simulink model "MultipleAgentsChoice_NoVR"  (Simulink 7.5)
settings: Solver=ode45  StartTime=0.0  StopTime=1000  RelTol=1e-4  AbsTol=1e-4
libraries: simulink x64
(part 2 of 6)

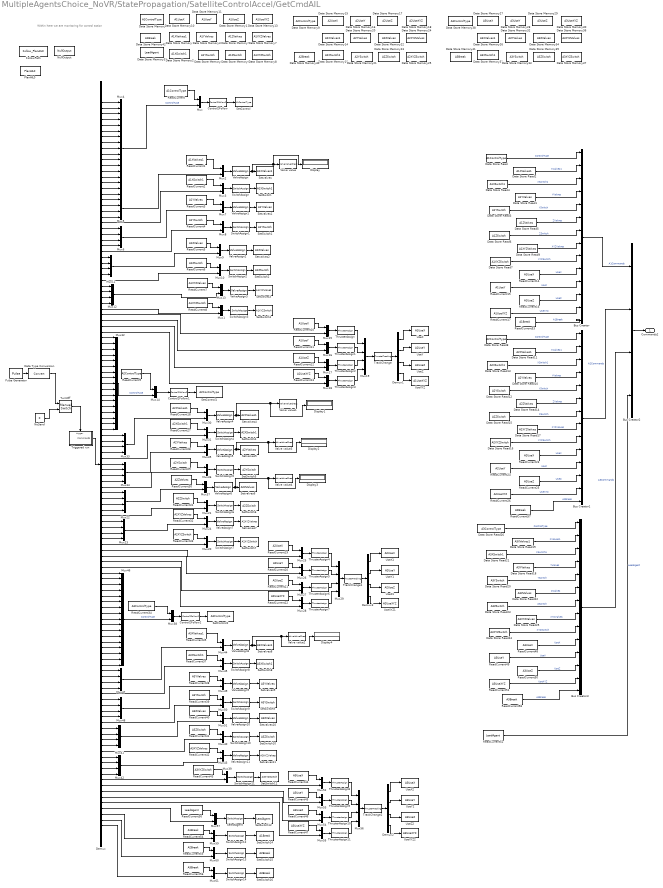
== system MultipleAgentsChoice_NoVR/StatePropagation/SatelliteControlAccel/GetCmdAIL ==
  note: Within here we are monitoring for control action
  Bus Creator : BusCreator  Inputs=14
  Bus Creator1 : BusCreator  Inputs=14
  Bus Creator2 : BusCreator
  Bus Creator3 : BusCreator  Inputs=14
  Control2Follow : MATLABFcn  MATLABFcn=Control2Follow2  OutputDimensions=17
  Control2Follow1 : MATLABFcn  MATLABFcn=Control2Follow2  OutputDimensions=17
  Control2Follow2 : MATLABFcn  MATLABFcn=Control2Follow2  OutputDimensions=17
  Data Store Memory : DataStoreMemory  DataStoreName=A1ControlType  ReadBeforeWriteMsg=warning  WriteAfterWriteMsg=warning  WriteAfterReadMsg=warning  InitialValue=[78;117;108;108;79;117;116;112;117;116;1;1;1;1;1;1;1]  OutDataType=sfix(16)  OutScaling=2^0
  Data Store Memory1 : DataStoreMemory  DataStoreName=A1XValves1  ReadBeforeWriteMsg=warning  WriteAfterWriteMsg=warning  WriteAfterReadMsg=warning  InitialValue=[2,2,1,1]  OutDataType=sfix(16)  OutScaling=2^0
  Data Store Memory10 : DataStoreMemory  DataStoreName=A1UseX  ReadBeforeWriteMsg=warning  WriteAfterWriteMsg=warning  WriteAfterReadMsg=warning  InitialValue=1  OutDataType=sfix(16)  OutScaling=2^0
  Data Store Memory11 : DataStoreMemory  DataStoreName=A1UseY  ReadBeforeWriteMsg=warning  WriteAfterWriteMsg=warning  WriteAfterReadMsg=warning  InitialValue=1  OutDataType=sfix(16)  OutScaling=2^0
  Data Store Memory12 : DataStoreMemory  DataStoreName=A1UseZ  ReadBeforeWriteMsg=warning  WriteAfterWriteMsg=warning  WriteAfterReadMsg=warning  InitialValue=1  OutDataType=sfix(16)  OutScaling=2^0
  Data Store Memory13 : DataStoreMemory  DataStoreName=A1UseXYZ  ReadBeforeWriteMsg=warning  WriteAfterWriteMsg=warning  WriteAfterReadMsg=warning  OutDataType=sfix(16)  OutScaling=2^0
  Data Store Memory14 : DataStoreMemory  DataStoreName=A2XValves1  ReadBeforeWriteMsg=warning  WriteAfterWriteMsg=warning  WriteAfterReadMsg=warning  InitialValue=[2,2,1,1]  OutDataType=sfix(16)  OutScaling=2^0
  Data Store Memory15 : DataStoreMemory  DataStoreName=A2UseX  ReadBeforeWriteMsg=warning  WriteAfterWriteMsg=warning  WriteAfterReadMsg=warning  InitialValue=1  OutDataType=sfix(16)  OutScaling=2^0
  Data Store Memory16 : DataStoreMemory  DataStoreName=A2UseY  ReadBeforeWriteMsg=warning  WriteAfterWriteMsg=warning  WriteAfterReadMsg=warning  InitialValue=1  OutDataType=sfix(16)  OutScaling=2^0
  Data Store Memory17 : DataStoreMemory  DataStoreName=A2UseZ  ReadBeforeWriteMsg=warning  WriteAfterWriteMsg=warning  WriteAfterReadMsg=warning  InitialValue=1  OutDataType=sfix(16)  OutScaling=2^0
  Data Store Memory18 : DataStoreMemory  DataStoreName=A2UseXYZ  ReadBeforeWriteMsg=warning  WriteAfterWriteMsg=warning  WriteAfterReadMsg=warning  OutDataType=sfix(16)  OutScaling=2^0
  Data Store Memory19 : DataStoreMemory  DataStoreName=A2XSwitch1  ReadBeforeWriteMsg=warning  WriteAfterWriteMsg=warning  WriteAfterReadMsg=warning  InitialValue=2  OutDataType=sfix(16)  OutScaling=2^0
  Data Store Memory2 : DataStoreMemory  DataStoreName=A1XSwitch1  ReadBeforeWriteMsg=warning  WriteAfterWriteMsg=warning  WriteAfterReadMsg=warning  InitialValue=2  OutDataType=sfix(16)  OutScaling=2^0
  Data Store Memory20 : DataStoreMemory  DataStoreName=A2YValves  ReadBeforeWriteMsg=warning  WriteAfterWriteMsg=warning  WriteAfterReadMsg=warning  InitialValue=[2,2,1,1]  OutDataType=sfix(16)  OutScaling=2^0
  Data Store Memory21 : DataStoreMemory  DataStoreName=A2YSwitch  ReadBeforeWriteMsg=warning  WriteAfterWriteMsg=warning  WriteAfterReadMsg=warning  InitialValue=2  OutDataType=sfix(16)  OutScaling=2^0
  Data Store Memory22 : DataStoreMemory  DataStoreName=A2ZValves  ReadBeforeWriteMsg=warning  WriteAfterWriteMsg=warning  WriteAfterReadMsg=warning  InitialValue=[2,2,1,1]  OutDataType=sfix(16)  OutScaling=2^0
  Data Store Memory23 : DataStoreMemory  DataStoreName=A2ZSwitch  ReadBeforeWriteMsg=warning  WriteAfterWriteMsg=warning  WriteAfterReadMsg=warning  InitialValue=2  OutDataType=sfix(16)  OutScaling=2^0
  Data Store Memory24 : DataStoreMemory  DataStoreName=A2XYZValves  ReadBeforeWriteMsg=warning  WriteAfterWriteMsg=warning  WriteAfterReadMsg=warning  InitialValue=[1,1,1,1]  OutDataType=sfix(16)  OutScaling=2^0
  Data Store Memory25 : DataStoreMemory  DataStoreName=A2XYZSwitch  ReadBeforeWriteMsg=warning  WriteAfterWriteMsg=warning  WriteAfterReadMsg=warning  InitialValue=1  OutDataType=sfix(16)  OutScaling=2^0
  Data Store Memory26 : DataStoreMemory  DataStoreName=A3XValves1  ReadBeforeWriteMsg=warning  WriteAfterWriteMsg=warning  WriteAfterReadMsg=warning  InitialValue=[2,2,1,1]  OutDataType=sfix(16)  OutScaling=2^0
  Data Store Memory27 : DataStoreMemory  DataStoreName=A3UseX  ReadBeforeWriteMsg=warning  WriteAfterWriteMsg=warning  WriteAfterReadMsg=warning  InitialValue=1  OutDataType=sfix(16)  OutScaling=2^0
  Data Store Memory28 : DataStoreMemory  DataStoreName=A3UseY  ReadBeforeWriteMsg=warning  WriteAfterWriteMsg=warning  WriteAfterReadMsg=warning  InitialValue=1  OutDataType=sfix(16)  OutScaling=2^0
  Data Store Memory29 : DataStoreMemory  DataStoreName=A3UseZ  ReadBeforeWriteMsg=warning  WriteAfterWriteMsg=warning  WriteAfterReadMsg=warning  InitialValue=1  OutDataType=sfix(16)  OutScaling=2^0
  Data Store Memory3 : DataStoreMemory  DataStoreName=A1YValves  ReadBeforeWriteMsg=warning  WriteAfterWriteMsg=warning  WriteAfterReadMsg=warning  InitialValue=[2,2,1,1]  OutDataType=sfix(16)  OutScaling=2^0
  Data Store Memory30 : DataStoreMemory  DataStoreName=A3UseXYZ  ReadBeforeWriteMsg=warning  WriteAfterWriteMsg=warning  WriteAfterReadMsg=warning  OutDataType=sfix(16)  OutScaling=2^0
  Data Store Memory31 : DataStoreMemory  DataStoreName=A3XSwitch1  ReadBeforeWriteMsg=warning  WriteAfterWriteMsg=warning  WriteAfterReadMsg=warning  InitialValue=2  OutDataType=sfix(16)  OutScaling=2^0
  Data Store Memory32 : DataStoreMemory  DataStoreName=A3YValves  ReadBeforeWriteMsg=warning  WriteAfterWriteMsg=warning  WriteAfterReadMsg=warning  InitialValue=[2,2,1,1]  OutDataType=sfix(16)  OutScaling=2^0
  Data Store Memory33 : DataStoreMemory  DataStoreName=A3YSwitch  ReadBeforeWriteMsg=warning  WriteAfterWriteMsg=warning  WriteAfterReadMsg=warning  InitialValue=2  OutDataType=sfix(16)  OutScaling=2^0
  Data Store Memory34 : DataStoreMemory  DataStoreName=A3ZValves  ReadBeforeWriteMsg=warning  WriteAfterWriteMsg=warning  WriteAfterReadMsg=warning  InitialValue=[2,2,1,1]  OutDataType=sfix(16)  OutScaling=2^0
  Data Store Memory35 : DataStoreMemory  DataStoreName=A3ZSwitch  ReadBeforeWriteMsg=warning  WriteAfterWriteMsg=warning  WriteAfterReadMsg=warning  InitialValue=2  OutDataType=sfix(16)  OutScaling=2^0
  Data Store Memory36 : DataStoreMemory  DataStoreName=A3XYZValves  ReadBeforeWriteMsg=warning  WriteAfterWriteMsg=warning  WriteAfterReadMsg=warning  InitialValue=[1,1,1,1]  OutDataType=sfix(16)  OutScaling=2^0
  Data Store Memory37 : DataStoreMemory  DataStoreName=A3XYZSwitch  ReadBeforeWriteMsg=warning  WriteAfterWriteMsg=warning  WriteAfterReadMsg=warning  InitialValue=1  OutDataType=sfix(16)  OutScaling=2^0
  Data Store Memory38 : DataStoreMemory  DataStoreName=A3ControlType  ReadBeforeWriteMsg=warning  WriteAfterWriteMsg=warning  WriteAfterReadMsg=warning  InitialValue=[78;117;108;108;79;117;116;112;117;116;1;1;1;1;1;1;1]  OutDataType=sfix(16)  OutScaling=2^0
  Data Store Memory39 : DataStoreMemory  DataStoreName=LeadAgent  ReadBeforeWriteMsg=warning  WriteAfterWriteMsg=warning  WriteAfterReadMsg=warning  InitialValue=1  OutDataType=sfix(16)  OutScaling=2^0
  Data Store Memory4 : DataStoreMemory  DataStoreName=A1YSwitch  ReadBeforeWriteMsg=warning  WriteAfterWriteMsg=warning  WriteAfterReadMsg=warning  InitialValue=2  OutDataType=sfix(16)  OutScaling=2^0
  Data Store Memory40 : DataStoreMemory  DataStoreName=A2Break  ReadBeforeWriteMsg=warning  WriteAfterWriteMsg=warning  WriteAfterReadMsg=warning  InitialValue=1  OutDataType=sfix(16)  OutScaling=2^0
  Data Store Memory41 : DataStoreMemory  DataStoreName=A3Break  ReadBeforeWriteMsg=warning  WriteAfterWriteMsg=warning  WriteAfterReadMsg=warning  InitialValue=1  OutDataType=sfix(16)  OutScaling=2^0
  Data Store Memory42 : DataStoreMemory  DataStoreName=A1Break  ReadBeforeWriteMsg=warning  WriteAfterWriteMsg=warning  WriteAfterReadMsg=warning  InitialValue=1  OutDataType=sfix(16)  OutScaling=2^0
  Data Store Memory5 : DataStoreMemory  DataStoreName=A1ZValves  ReadBeforeWriteMsg=warning  WriteAfterWriteMsg=warning  WriteAfterReadMsg=warning  InitialValue=[2,2,1,1]  OutDataType=sfix(16)  OutScaling=2^0
  Data Store Memory6 : DataStoreMemory  DataStoreName=A1ZSwitch  ReadBeforeWriteMsg=warning  WriteAfterWriteMsg=warning  WriteAfterReadMsg=warning  InitialValue=2  OutDataType=sfix(16)  OutScaling=2^0
  Data Store Memory7 : DataStoreMemory  DataStoreName=A1XYZValves  ReadBeforeWriteMsg=warning  WriteAfterWriteMsg=warning  WriteAfterReadMsg=warning  InitialValue=[1,1,1,1]  OutDataType=sfix(16)  OutScaling=2^0
  Data Store Memory8 : DataStoreMemory  DataStoreName=A1XYZSwitch  ReadBeforeWriteMsg=warning  WriteAfterWriteMsg=warning  WriteAfterReadMsg=warning  InitialValue=1  OutDataType=sfix(16)  OutScaling=2^0
  Data Store Memory9 : DataStoreMemory  DataStoreName=A2ControlType  ReadBeforeWriteMsg=warning  WriteAfterWriteMsg=warning  WriteAfterReadMsg=warning  InitialValue=[78;117;108;108;79;117;116;112;117;116;1;1;1;1;1;1;1]  OutDataType=sfix(16)  OutScaling=2^0
  Data Store Read : DataStoreRead  DataStoreName=A1ControlType  SampleTime=-1
  Data Store Read1 : DataStoreRead  DataStoreName=A1YValves  SampleTime=-1
  Data Store Read10 : DataStoreRead  DataStoreName=A2YValves  SampleTime=-1
  Data Store Read11 : DataStoreRead  DataStoreName=A2XValves1  SampleTime=-1
  Data Store Read12 : DataStoreRead  DataStoreName=A2YSwitch  SampleTime=-1
  Data Store Read13 : DataStoreRead  DataStoreName=A2XSwitch1  SampleTime=-1
  Data Store Read14 : DataStoreRead  DataStoreName=A2ZValves  SampleTime=-1
  Data Store Read15 : DataStoreRead  DataStoreName=A2ZSwitch  SampleTime=-1
  Data Store Read16 : DataStoreRead  DataStoreName=A2XYZSwitch  SampleTime=-1
  Data Store Read17 : DataStoreRead  DataStoreName=A2XYZValves  SampleTime=-1
  Data Store Read18 : DataStoreRead  DataStoreName=A3YValves  SampleTime=-1
  Data Store Read19 : DataStoreRead  DataStoreName=A3XValves1  SampleTime=-1
  Data Store Read2 : DataStoreRead  DataStoreName=A1XValves1  SampleTime=-1
  Data Store Read20 : DataStoreRead  DataStoreName=A3YSwitch  SampleTime=-1
  Data Store Read21 : DataStoreRead  DataStoreName=A3XSwitch1  SampleTime=-1
  Data Store Read22 : DataStoreRead  DataStoreName=A3ZValves  SampleTime=-1
  Data Store Read23 : DataStoreRead  DataStoreName=A3ZSwitch  SampleTime=-1
  Data Store Read24 : DataStoreRead  DataStoreName=A3XYZSwitch  SampleTime=-1
  Data Store Read25 : DataStoreRead  DataStoreName=A3XYZValves  SampleTime=-1
  Data Store Read26 : DataStoreRead  DataStoreName=A3ControlType  SampleTime=-1
  Data Store Read3 : DataStoreRead  DataStoreName=A1YSwitch  SampleTime=-1
  Data Store Read4 : DataStoreRead  DataStoreName=A1XSwitch1  SampleTime=-1
  Data Store Read5 : DataStoreRead  DataStoreName=A1ZValves  SampleTime=-1
  Data Store Read6 : DataStoreRead  DataStoreName=A1ZSwitch  SampleTime=-1
  Data Store Read7 : DataStoreRead  DataStoreName=A1XYZSwitch  SampleTime=-1
  Data Store Read8 : DataStoreRead  DataStoreName=A2ControlType  SampleTime=-1
  Data Store Read9 : DataStoreRead  DataStoreName=A1XYZValves  SampleTime=-1
  Data Type Conversion : DataTypeConversion  OutDataType=sfix(16)  OutScaling=2^0
  Demux : Demux  Outputs=127
  Demux1 : Demux
  Demux2 : Demux
  Demux3 : Demux
  Display{,1..4} (5 alike) : Display
  FollowPath : DataStoreMemory  DataStoreName=Follow_PlanAIL0  ReadBeforeWriteMsg=warning  WriteAfterWriteMsg=warning  WriteAfterReadMsg=warning  InitialValue=[70;111;108;108;111;119 ;32;80;108;97;110;65;73;76;48;1;1]  OutDataType=sfix(16)  OutScaling=2^0
  Mux{,1..3,7..10,13..18,20..21,24..28,30..31,35..40,43..45,49..55,57,59..61} (43 alike) : Mux  Inputs=2
  Mux{5..6,11..12,19,22..23,29,33..34,41..42,47..48,56} (15 alike) : Mux
  Mux32 : Mux  Inputs=17
  Mux4 : Mux  Inputs=17
  Mux46 : Mux  Inputs=17
  NoSend : Constant  Value=0  OutDataType=sfix(16)  OutScaling=2^0
  NullOutput : DataStoreMemory  DataStoreName=NullOutput  ReadBeforeWriteMsg=warning  WriteAfterWriteMsg=warning  WriteAfterReadMsg=warning  InitialValue=[78;117;108;108;79;117;116;112;117;116;1;1;1;1;1;1;1]  OutDataType=sfix(16)  OutScaling=2^0
  PlanAIL0 : DataStoreMemory  DataStoreName=PlanAIL0  ReadBeforeWriteMsg=warning  WriteAfterWriteMsg=warning  WriteAfterReadMsg=warning  InitialValue=[80;108;97;110;65;73 ;76; 48;1;1; 1;1 ;1;1;1;1;1]  OutDataType=sfix(16)  OutScaling=2^0
  Pulse Generator : DiscretePulseGenerator  PulseType=Time based  Amplitude=1  Period=0.1  PulseWidth=50  PhaseDelay=0  SampleTime=1
  ReadCurrent : DataStoreRead  DataStoreName=A1ControlType  SampleTime=-1
  ReadCurrent1 : DataStoreRead  DataStoreName=A1XValves1  SampleTime=-1
  ReadCurrent10 : DataStoreRead  DataStoreName=A1UseX  SampleTime=-1
  ReadCurrent11 : DataStoreRead  DataStoreName=A1UseY  SampleTime=-1
  ReadCurrent12 : DataStoreRead  DataStoreName=A1UseZ  SampleTime=-1
  ReadCurrent13 : DataStoreRead  DataStoreName=A1UseXYZ  SampleTime=-1
  ReadCurrent14 : DataStoreRead  DataStoreName=A1UseX  SampleTime=-1
  ReadCurrent15 : DataStoreRead  DataStoreName=A1UseY  SampleTime=-1
  ReadCurrent16 : DataStoreRead  DataStoreName=A1UseZ  SampleTime=-1
  ReadCurrent17 : DataStoreRead  DataStoreName=A1UseXYZ  SampleTime=-1
  ReadCurrent18 : DataStoreRead  DataStoreName=A2XValves1  SampleTime=-1
  ReadCurrent19 : DataStoreRead  DataStoreName=A2UseX  SampleTime=-1
  ReadCurrent2 : DataStoreRead  DataStoreName=A1XSwitch1  SampleTime=-1
  ReadCurrent20 : DataStoreRead  DataStoreName=A2UseY  SampleTime=-1
  ReadCurrent21 : DataStoreRead  DataStoreName=A2UseZ  SampleTime=-1
  ReadCurrent22 : DataStoreRead  DataStoreName=A2UseXYZ  SampleTime=-1
  ReadCurrent23 : DataStoreRead  DataStoreName=A2UseX  SampleTime=-1
  ReadCurrent24 : DataStoreRead  DataStoreName=A2UseY  SampleTime=-1
  ReadCurrent25 : DataStoreRead  DataStoreName=A2UseZ  SampleTime=-1
  ReadCurrent26 : DataStoreRead  DataStoreName=A2UseXYZ  SampleTime=-1
  ReadCurrent27 : DataStoreRead  DataStoreName=A2XSwitch1  SampleTime=-1
  ReadCurrent28 : DataStoreRead  DataStoreName=A2YValves  SampleTime=-1
  ReadCurrent29 : DataStoreRead  DataStoreName=A2YSwitch  SampleTime=-1
  ReadCurrent3 : DataStoreRead  DataStoreName=A1YValves  SampleTime=-1
  ReadCurrent30 : DataStoreRead  DataStoreName=A2ZValves  SampleTime=-1
  ReadCurrent31 : DataStoreRead  DataStoreName=A2ZSwitch  SampleTime=-1
  ReadCurrent32 : DataStoreRead  DataStoreName=A2XYZValves  SampleTime=-1
  ReadCurrent33 : DataStoreRead  DataStoreName=A2XYZSwitch  SampleTime=-1
  ReadCurrent34 : DataStoreRead  DataStoreName=A3ControlType  SampleTime=-1
  ReadCurrent35 : DataStoreRead  DataStoreName=A3XValves1  SampleTime=-1
  ReadCurrent36 : DataStoreRead  DataStoreName=LeadAgent  SampleTime=-1
  ReadCurrent37 : DataStoreRead  DataStoreName=A3XSwitch1  SampleTime=-1
  ReadCurrent38 : DataStoreRead  DataStoreName=A3YValves  SampleTime=-1
  ReadCurrent39 : DataStoreRead  DataStoreName=A3YSwitch  SampleTime=-1
  ReadCurrent4 : DataStoreRead  DataStoreName=A1YSwitch  SampleTime=-1
  ReadCurrent40 : DataStoreRead  DataStoreName=A3ZValves  SampleTime=-1
  ReadCurrent41 : DataStoreRead  DataStoreName=A3ZSwitch  SampleTime=-1
  ReadCurrent42 : DataStoreRead  DataStoreName=A3XYZValves  SampleTime=-1
  ReadCurrent43 : DataStoreRead  DataStoreName=A3XYZSwitch  SampleTime=-1
  ReadCurrent44 : DataStoreRead  DataStoreName=A3UseX  SampleTime=-1
  ReadCurrent45 : DataStoreRead  DataStoreName=A3UseY  SampleTime=-1
  ReadCurrent46 : DataStoreRead  DataStoreName=A3UseZ  SampleTime=-1
  ReadCurrent47 : DataStoreRead  DataStoreName=A3UseXYZ  SampleTime=-1
  ReadCurrent48 : DataStoreRead  DataStoreName=A3UseX  SampleTime=-1
  ReadCurrent49 : DataStoreRead  DataStoreName=A3UseY  SampleTime=-1
  ReadCurrent5 : DataStoreRead  DataStoreName=A1ZValves  SampleTime=-1
  ReadCurrent50 : DataStoreRead  DataStoreName=A3UseZ  SampleTime=-1
  ReadCurrent51 : DataStoreRead  DataStoreName=A3UseXYZ  SampleTime=-1
  ReadCurrent52 : DataStoreRead  DataStoreName=LeadAgent  SampleTime=-1
  ReadCurrent53 : DataStoreRead  DataStoreName=A1Break  SampleTime=-1
  ReadCurrent54 : DataStoreRead  DataStoreName=A1Break  SampleTime=-1
  ReadCurrent55 : DataStoreRead  DataStoreName=A2Break  SampleTime=-1
  ReadCurrent56 : DataStoreRead  DataStoreName=A3Break  SampleTime=-1
  ReadCurrent57 : DataStoreRead  DataStoreName=A2Break  SampleTime=-1
  ReadCurrent58 : DataStoreRead  DataStoreName=A3Break  SampleTime=-1
  ReadCurrent6 : DataStoreRead  DataStoreName=A1ZSwitch  SampleTime=-1
  ReadCurrent7 : DataStoreRead  DataStoreName=A1XYZValves  SampleTime=-1
  ReadCurrent8 : DataStoreRead  DataStoreName=A1XYZSwitch  SampleTime=-1
  ReadCurrent9 : DataStoreRead  DataStoreName=A2ControlType  SampleTime=-1
  SelectAgent : MATLABFcn  MATLABFcn=SwitchAssign  OutputDimensions=1
  SetControl : DataStoreWrite  DataStoreName=A1ControlType  SampleTime=-1
  SetControl1 : DataStoreWrite  DataStoreName=A2ControlType  SampleTime=-1
  SetControl2 : DataStoreWrite  DataStoreName=A3ControlType  SampleTime=-1
  SetSwitch : DataStoreWrite  DataStoreName=A1XSwitch1  SampleTime=-1
  SetSwitch1 : DataStoreWrite  DataStoreName=A1YSwitch  SampleTime=-1
  SetSwitch10 : DataStoreWrite  DataStoreName=A3ZSwitch  SampleTime=-1
  SetSwitch11 : DataStoreWrite  DataStoreName=A3XYZSwitch  SampleTime=-1
  SetSwitch12 : DataStoreWrite  DataStoreName=LeadAgent  SampleTime=-1
  SetSwitch14 : DataStoreWrite  DataStoreName=A1Break  SampleTime=-1
  SetSwitch15 : DataStoreWrite  DataStoreName=A2Break  SampleTime=-1
  SetSwitch16 : DataStoreWrite  DataStoreName=A3Break  SampleTime=-1
  SetSwitch2 : DataStoreWrite  DataStoreName=A1ZSwitch  SampleTime=-1
  SetSwitch3 : DataStoreWrite  DataStoreName=A1XYZSwitch  SampleTime=-1
  SetSwitch4 : DataStoreWrite  DataStoreName=A2XSwitch1  SampleTime=-1
  SetSwitch5 : DataStoreWrite  DataStoreName=A2YSwitch  SampleTime=-1
  SetSwitch6 : DataStoreWrite  DataStoreName=A2ZSwitch  SampleTime=-1
  SetSwitch7 : DataStoreWrite  DataStoreName=A2XYZSwitch  SampleTime=-1
  SetSwitch8 : DataStoreWrite  DataStoreName=A3XSwitch1  SampleTime=-1
  SetSwitch9 : DataStoreWrite  DataStoreName=A3YSwitch  SampleTime=-1
  Setvalves : DataStoreWrite  DataStoreName=A1XValves1  SampleTime=-1
  Setvalves1 : DataStoreWrite  DataStoreName=A1YValves  SampleTime=-1
  Setvalves10 : DataStoreWrite  DataStoreName=A3ZValves  SampleTime=-1
  Setvalves11 : DataStoreWrite  DataStoreName=A3XYZValves  SampleTime=-1
  Setvalves2 : DataStoreWrite  DataStoreName=A1ZValves  SampleTime=-1
  Setvalves3 : DataStoreWrite  DataStoreName=A1XYZValves  SampleTime=-1
  Setvalves4 : DataStoreWrite  DataStoreName=A2XValves1  SampleTime=-1
  Setvalves5 : DataStoreWrite  DataStoreName=A2YValves  SampleTime=-1
  Setvalves6 : DataStoreWrite  DataStoreName=A2ZValves  SampleTime=-1
  Setvalves7 : DataStoreWrite  DataStoreName=A2XYZValves  SampleTime=-1
  Setvalves8 : DataStoreWrite  DataStoreName=A3XValves1  SampleTime=-1
  Setvalves9 : DataStoreWrite  DataStoreName=A3YValves  SampleTime=-1
  SwitchAssign{,1..14} (15 alike) : MATLABFcn  MATLABFcn=SwitchAssign  OutputDimensions=1
  ThrusterAssign{,1..11} (12 alike) : MATLABFcn  MATLABFcn=ThrusterAssign  OutputDimensions=1
  TrackChange : MATLABFcn  MATLABFcn=ThrusterTracking  OutputDimensions=4
  TrackChange1 : MATLABFcn  MATLABFcn=ThrusterTracking  OutputDimensions=4
  TrackChange2 : MATLABFcn  MATLABFcn=ThrusterTracking  OutputDimensions=4
  Triggered run : Subsystem  TreatAsAtomicUnit=on
  TurnOff : simulink/Signal Routing/Manual Switch  SystemSampleTime=-1  sw=1  action=0  varsize=off
  UseX : DataStoreWrite  DataStoreName=A1UseX  SampleTime=-1
  UseX1 : DataStoreWrite  DataStoreName=A2UseX  SampleTime=-1
  UseX2 : DataStoreWrite  DataStoreName=A3UseX  SampleTime=-1
  UseXYZ : DataStoreWrite  DataStoreName=A1UseXYZ  SampleTime=-1
  UseXYZ1 : DataStoreWrite  DataStoreName=A2UseXYZ  SampleTime=-1
  UseXYZ2 : DataStoreWrite  DataStoreName=A3UseXYZ  SampleTime=-1
  UseY : DataStoreWrite  DataStoreName=A1UseY  SampleTime=-1
  UseY1 : DataStoreWrite  DataStoreName=A2UseY  SampleTime=-1
  UseY2 : DataStoreWrite  DataStoreName=A3UseY  SampleTime=-1
  UseZ : DataStoreWrite  DataStoreName=A1UseZ  SampleTime=-1
  UseZ1 : DataStoreWrite  DataStoreName=A2UseZ  SampleTime=-1
  UseZ2 : DataStoreWrite  DataStoreName=A3UseZ  SampleTime=-1
  Valve value{,1..4} (5 alike) : MATLABFcn  MATLABFcn=ValveValueCheck  OutputDimensions=0
  ValveAssign{,1..11} (12 alike) : MATLABFcn  MATLABFcn=ValveAssign  OutputDimensions=4
  Commands2 : Outport  OutDataType=sfix(16)  OutScaling=2^0
  wires:
  Pulse Generator/1 -> Data Type Conversion/1
  Data Store Read/1 -> Bus Creator/1  "ControlType"
  Data Store Read2/1 -> Bus Creator/2  "XValves1"
  Mux2/1 -> ValveAssign/1
  ValveAssign/1 -> Setvalves/1, Valve value/1, Display/1
  ReadCurrent1/1 -> Mux2/1
  Data Store Read4/1 -> Bus Creator/3  "XSwitch1"
  Mux3/1 -> SwitchAssign/1
  SwitchAssign/1 -> SetSwitch/1
  ReadCurrent2/1 -> Mux3/1
  Bus Creator/1 -> Bus Creator2/1  "A1Commands"
  Triggered run/1(Commands) -> Demux/1
  Control2Follow/1 -> SetControl/1
  Mux/1 -> Control2Follow/1
  ReadCurrent/1 -> Mux/1
  Mux4/1 -> Mux/2  "ControlType"
  Data Store Read1/1 -> Bus Creator/4  "YValves"
  Data Store Read3/1 -> Bus Creator/5  "YSwitch"
  Data Store Read5/1 -> Bus Creator/6  "ZValves"
  Data Store Read6/1 -> Bus Creator/7  "ZSwitch"
  Mux7/1 -> ValveAssign1/1
  ValveAssign1/1 -> Setvalves1/1
  ReadCurrent3/1 -> Mux7/1
  Mux8/1 -> SwitchAssign1/1
  SwitchAssign1/1 -> SetSwitch1/1
  ReadCurrent4/1 -> Mux8/1
  Mux9/1 -> ValveAssign2/1
  ValveAssign2/1 -> Setvalves2/1
  ReadCurrent5/1 -> Mux9/1
  Mux10/1 -> SwitchAssign2/1
  SwitchAssign2/1 -> SetSwitch2/1
  ReadCurrent6/1 -> Mux10/1
  TurnOff/1 -> Triggered run/Trigger
  Data Type Conversion/1 -> TurnOff/1
  NoSend/1 -> TurnOff/2
  Mux5/1 -> Mux2/2
  Mux6/1 -> Mux7/2
  Mux11/1 -> Mux9/2
  Mux13/1 -> ValveAssign3/1
  ValveAssign3/1 -> Setvalves3/1
  ReadCurrent7/1 -> Mux13/1
  Mux1/1 -> SwitchAssign3/1
  SwitchAssign3/1 -> SetSwitch3/1
  ReadCurrent8/1 -> Mux1/1
  Mux12/1 -> Mux13/2
  Data Store Read9/1 -> Bus Creator/8  "XYZValves"
  Data Store Read7/1 -> Bus Creator/9  "XYZSwitch"
  Mux15/1 -> ThrusterAssign/1
  ReadCurrent10/1 -> Mux15/1
  Mux16/1 -> ThrusterAssign1/1
  ReadCurrent11/1 -> Mux16/1
  Mux17/1 -> ThrusterAssign2/1
  ReadCurrent12/1 -> Mux17/1
  Mux18/1 -> ThrusterAssign3/1
  ReadCurrent13/1 -> Mux18/1
  ReadCurrent14/1 -> Bus Creator/10  "UseX"
  ReadCurrent15/1 -> Bus Creator/11  "UseY"
  ReadCurrent16/1 -> Bus Creator/12  "UseZ"
  ReadCurrent17/1 -> Bus Creator/13  "UseXYZ"
  ThrusterAssign1/1 -> Mux19/2
  ThrusterAssign2/1 -> Mux19/3
  ThrusterAssign3/1 -> Mux19/4
  ThrusterAssign/1 -> Mux19/1
  Mux19/1 -> TrackChange/1
  TrackChange/1 -> Demux1/1
  Demux1/1 -> UseX/1
  Demux1/2 -> UseY/1
  Demux1/3 -> UseZ/1
  Demux1/4 -> UseXYZ/1
  Data Store Read8/1 -> Bus Creator1/1  "ControlType"
  Data Store Read11/1 -> Bus Creator1/2  "XValves1"
  Mux30/1 -> ValveAssign4/1
  ValveAssign4/1 -> Setvalves4/1, Valve value1/1, Display1/1
  ReadCurrent18/1 -> Mux30/1
  Data Store Read13/1 -> Bus Creator1/3  "XSwitch1"
  Mux31/1 -> SwitchAssign4/1
  SwitchAssign4/1 -> SetSwitch4/1
  ReadCurrent27/1 -> Mux31/1
  Bus Creator1/1 -> Bus Creator2/2  "A2Commands"
  Control2Follow1/1 -> SetControl1/1
  Mux14/1 -> Control2Follow1/1
  ReadCurrent9/1 -> Mux14/1
  Mux32/1 -> Mux14/2  "ControlType"
  Data Store Read10/1 -> Bus Creator1/4  "YValves"
  Data Store Read12/1 -> Bus Creator1/5  "YSwitch"
  Data Store Read14/1 -> Bus Creator1/6  "ZValves"
  Data Store Read15/1 -> Bus Creator1/7  "ZSwitch"
  Mux35/1 -> ValveAssign5/1
  ValveAssign5/1 -> Setvalves5/1, Valve value3/1, Display2/1
  ReadCurrent28/1 -> Mux35/1
  Mux36/1 -> SwitchAssign5/1
  SwitchAssign5/1 -> SetSwitch5/1
  ReadCurrent29/1 -> Mux36/1
  Mux37/1 -> ValveAssign6/1
  ValveAssign6/1 -> Setvalves6/1, Valve value4/1, Display3/1
  ReadCurrent30/1 -> Mux37/1
  Mux21/1 -> SwitchAssign6/1
  SwitchAssign6/1 -> SetSwitch6/1
  ReadCurrent31/1 -> Mux21/1
  Mux33/1 -> Mux30/2
  Mux34/1 -> Mux35/2
  Mux22/1 -> Mux37/2
  Mux24/1 -> ValveAssign7/1
  ValveAssign7/1 -> Setvalves7/1
  ReadCurrent32/1 -> Mux24/1
  Mux20/1 -> SwitchAssign7/1
  SwitchAssign7/1 -> SetSwitch7/1
  ReadCurrent33/1 -> Mux20/1
  Mux23/1 -> Mux24/2
  Data Store Read17/1 -> Bus Creator1/8  "XYZValves"
  Data Store Read16/1 -> Bus Creator1/9  "XYZSwitch"
  Mux25/1 -> ThrusterAssign4/1
  ReadCurrent19/1 -> Mux25/1
  Mux26/1 -> ThrusterAssign5/1
  ReadCurrent20/1 -> Mux26/1
  Mux27/1 -> ThrusterAssign6/1
  ReadCurrent21/1 -> Mux27/1
  Mux28/1 -> ThrusterAssign7/1
  ReadCurrent22/1 -> Mux28/1
  ReadCurrent23/1 -> Bus Creator1/10  "UseX"
  ReadCurrent24/1 -> Bus Creator1/11  "UseY"
  ReadCurrent25/1 -> Bus Creator1/12  "UseZ"
  ReadCurrent26/1 -> Bus Creator1/13  "UseXYZ"
  ThrusterAssign5/1 -> Mux29/2
  ThrusterAssign6/1 -> Mux29/3
  ThrusterAssign7/1 -> Mux29/4
  ThrusterAssign4/1 -> Mux29/1
  Mux29/1 -> TrackChange1/1
  TrackChange1/1 -> Demux3/1
  Demux3/1 -> UseX1/1
  Demux3/2 -> UseY1/1
  Demux3/3 -> UseZ1/1
  Demux3/4 -> UseXYZ1/1
  Bus Creator2/1 -> Commands2/1
  Mux44/1 -> ValveAssign8/1
  ValveAssign8/1 -> Setvalves8/1, Valve value2/1, Display4/1
  ReadCurrent35/1 -> Mux44/1
  Mux45/1 -> SwitchAssign8/1
  SwitchAssign8/1 -> SetSwitch8/1
  ReadCurrent37/1 -> Mux45/1
  Control2Follow2/1 -> SetControl2/1
  Mux38/1 -> Control2Follow2/1
  ReadCurrent34/1 -> Mux38/1
  Mux46/1 -> Mux38/2  "ControlType"
  Mux49/1 -> ValveAssign9/1
  ValveAssign9/1 -> Setvalves9/1
  ReadCurrent38/1 -> Mux49/1
  Mux50/1 -> SwitchAssign9/1
  SwitchAssign9/1 -> SetSwitch9/1
  ReadCurrent39/1 -> Mux50/1
  Mux51/1 -> ValveAssign10/1
  ValveAssign10/1 -> Setvalves10/1
  ReadCurrent40/1 -> Mux51/1
  Mux40/1 -> SwitchAssign10/1
  SwitchAssign10/1 -> SetSwitch10/1
  ReadCurrent41/1 -> Mux40/1
  Mux47/1 -> Mux44/2
  Mux48/1 -> Mux49/2
  Mux41/1 -> Mux51/2
  Mux43/1 -> ValveAssign11/1
  ValveAssign11/1 -> Setvalves11/1
  ReadCurrent42/1 -> Mux43/1
  Mux39/1 -> SwitchAssign11/1
  SwitchAssign11/1 -> SetSwitch11/1
  ReadCurrent43/1 -> Mux39/1
  Mux42/1 -> Mux43/2
  Mux52/1 -> ThrusterAssign8/1
  ReadCurrent44/1 -> Mux52/1
  Mux53/1 -> ThrusterAssign9/1
  ReadCurrent45/1 -> Mux53/1
  Mux54/1 -> ThrusterAssign10/1
  ReadCurrent46/1 -> Mux54/1
  Mux55/1 -> ThrusterAssign11/1
  ReadCurrent47/1 -> Mux55/1
  ThrusterAssign9/1 -> Mux56/2
  ThrusterAssign10/1 -> Mux56/3
  ThrusterAssign11/1 -> Mux56/4
  ThrusterAssign8/1 -> Mux56/1
  Mux56/1 -> TrackChange2/1
  TrackChange2/1 -> Demux2/1
  Demux2/1 -> UseX2/1
  Demux2/2 -> UseY2/1
  Demux2/3 -> UseZ2/1
  Demux2/4 -> UseXYZ2/1
  ReadCurrent36/1 -> Mux57/1
  Mux57/1 -> SelectAgent/1
  SelectAgent/1 -> SetSwitch12/1
  Data Store Read26/1 -> Bus Creator3/1  "ControlType"
  Data Store Read19/1 -> Bus Creator3/2  "XValves1"
  Data Store Read21/1 -> Bus Creator3/3  "XSwitch1"
  Data Store Read18/1 -> Bus Creator3/4  "YValves"
  Data Store Read20/1 -> Bus Creator3/5  "YSwitch"
  Data Store Read22/1 -> Bus Creator3/6  "ZValves"
  Data Store Read23/1 -> Bus Creator3/7  "ZSwitch"
  Data Store Read25/1 -> Bus Creator3/8  "XYZValves"
  Data Store Read24/1 -> Bus Creator3/9  "XYZSwitch"
  ReadCurrent48/1 -> Bus Creator3/10  "UseX"
  ReadCurrent49/1 -> Bus Creator3/11  "UseY"
  ReadCurrent50/1 -> Bus Creator3/12  "UseZ"
  ReadCurrent51/1 -> Bus Creator3/13  "UseXYZ"
  Bus Creator3/1 -> Bus Creator2/3  "A3Commands"
  ReadCurrent52/1 -> Bus Creator2/4  "LeadAgent"
  Demux/124 -> Mux57/2
  Demux/123 -> Mux55/2
  Demux/122 -> Mux54/2
  Demux/121 -> Mux53/2
  Demux/120 -> Mux52/2
  Demux/119 -> Mux39/2
  Demux/115 -> Mux42/1
  Demux/116 -> Mux42/2
  Demux/117 -> Mux42/3
  Demux/118 -> Mux42/4
  Demux/114 -> Mux40/2
  Demux/110 -> Mux41/1
  Demux/111 -> Mux41/2
  Demux/112 -> Mux41/3
  Demux/113 -> Mux41/4
  Demux/109 -> Mux50/2
  Demux/105 -> Mux48/1
  Demux/106 -> Mux48/2
  Demux/107 -> Mux48/3
  Demux/108 -> Mux48/4
  Demux/104 -> Mux45/2
  Demux/100 -> Mux47/1
  Demux/101 -> Mux47/2
  Demux/102 -> Mux47/3
  Demux/103 -> Mux47/4
  Demux/99 -> Mux46/17
  Demux/98 -> Mux46/16
  Demux/97 -> Mux46/15
  Demux/96 -> Mux46/14
  Demux/95 -> Mux46/13
  Demux/94 -> Mux46/12
  Demux/93 -> Mux46/11
  Demux/83 -> Mux46/1
  Demux/84 -> Mux46/2
  Demux/85 -> Mux46/3
  Demux/86 -> Mux46/4
  Demux/87 -> Mux46/5
  Demux/88 -> Mux46/6
  Demux/89 -> Mux46/7
  Demux/90 -> Mux46/8
  Demux/91 -> Mux46/9
  Demux/92 -> Mux46/10
  Demux/82 -> Mux28/2
  Demux/81 -> Mux27/2
  Demux/80 -> Mux26/2
  Demux/79 -> Mux25/2
  Demux/78 -> Mux20/2
  Demux/74 -> Mux23/1
  Demux/75 -> Mux23/2
  Demux/76 -> Mux23/3
  Demux/77 -> Mux23/4
  Demux/1 -> Mux4/1
  Demux/2 -> Mux4/2
  Demux/3 -> Mux4/3
  Demux/4 -> Mux4/4
  Demux/5 -> Mux4/5
  Demux/6 -> Mux4/6
  Demux/7 -> Mux4/7
  Demux/8 -> Mux4/8
  Demux/9 -> Mux4/9
  Demux/10 -> Mux4/10
  Demux/11 -> Mux4/11
  Demux/12 -> Mux4/12
  Demux/13 -> Mux4/13
  Demux/14 -> Mux4/14
  Demux/15 -> Mux4/15
  Demux/16 -> Mux4/16
  Demux/17 -> Mux4/17
  Demux/18 -> Mux5/1
  Demux/19 -> Mux5/2
  Demux/20 -> Mux5/3
  Demux/21 -> Mux5/4
  Demux/22 -> Mux3/2
  Demux/23 -> Mux6/1
  Demux/24 -> Mux6/2
  Demux/25 -> Mux6/3
  Demux/26 -> Mux6/4
  Demux/27 -> Mux8/2
  Demux/28 -> Mux11/1
  Demux/29 -> Mux11/2
  Demux/30 -> Mux11/3
  Demux/31 -> Mux11/4
  Demux/32 -> Mux10/2
  Demux/33 -> Mux12/1
  Demux/34 -> Mux12/2
  Demux/35 -> Mux12/3
  Demux/36 -> Mux12/4
  Demux/37 -> Mux1/2
  Demux/38 -> Mux15/2
  Demux/39 -> Mux16/2
  Demux/40 -> Mux17/2
  Demux/41 -> Mux18/2
  Demux/42 -> Mux32/1
  Demux/43 -> Mux32/2
  Demux/44 -> Mux32/3
  Demux/45 -> Mux32/4
  Demux/46 -> Mux32/5
  Demux/47 -> Mux32/6
  Demux/48 -> Mux32/7
  Demux/49 -> Mux32/8
  Demux/50 -> Mux32/9
  Demux/51 -> Mux32/10
  Demux/52 -> Mux32/11
  Demux/53 -> Mux32/12
  Demux/54 -> Mux32/13
  Demux/55 -> Mux32/14
  Demux/56 -> Mux32/15
  Demux/57 -> Mux32/16
  Demux/58 -> Mux32/17
  Demux/59 -> Mux33/1
  Demux/60 -> Mux33/2
  Demux/61 -> Mux33/3
  Demux/62 -> Mux33/4
  Demux/63 -> Mux31/2
  Demux/64 -> Mux34/1
  Demux/65 -> Mux34/2
  Demux/66 -> Mux34/3
  Demux/67 -> Mux34/4
  Demux/68 -> Mux36/2
  Demux/69 -> Mux22/1
  Demux/70 -> Mux22/2
  Demux/71 -> Mux22/3
  Demux/72 -> Mux22/4
  Demux/73 -> Mux21/2
  Demux/125 -> Mux59/2
  Demux/126 -> Mux60/2
  Demux/127 -> Mux61/2
  Mux59/1 -> SwitchAssign12/1
  ReadCurrent54/1 -> Mux59/1
  SwitchAssign12/1 -> SetSwitch14/1
  ReadCurrent55/1 -> Mux60/1
  ReadCurrent56/1 -> Mux61/1
  Mux60/1 -> SwitchAssign13/1
  SwitchAssign13/1 -> SetSwitch15/1
  SwitchAssign14/1 -> SetSwitch16/1
  Mux61/1 -> SwitchAssign14/1
  ReadCurrent58/1 -> Bus Creator3/14  "A3Break"
  ReadCurrent53/1 -> Bus Creator/14  "A1Break"
  ReadCurrent57/1 -> Bus Creator1/14  "A2Break"

== system MultipleAgentsChoice_NoVR/StatePropagation/SatelliteControlAccel/InitialErrors ==
  A1PosVelDiff : Constant  Value=[0.05;0.05;0;0;0;0]  OutDataType=sfix(16)  OutScaling=2^0
  A2PosVelDiff : Constant  Value=[-0.05;0;-0.05;0;0;0];  OutDataType=sfix(16)  OutScaling=2^0
  Altitude(km) Eccentricity : Constant  Value=[400;0]  OutDataType=sfix(16)  OutScaling=2^0
  Bus Creator : BusCreator  Inputs=3
  StartIdeal : MATLABFcn  MATLABFcn=StartIdeal  OutputDimensions=6
  Sum : Sum  Inputs=|++  OutDataType=sfix(16)  OutScaling=2^0
  Sum1 : Sum  Inputs=|++  OutDataType=sfix(16)  OutScaling=2^0
  Out1 : Outport  OutDataType=sfix(16)  OutScaling=2^0
  wires:
  A1PosVelDiff/1 -> Sum/1
  A2PosVelDiff/1 -> Sum1/1
  Sum/1 -> Bus Creator/1  "Agent1"
  Sum1/1 -> Bus Creator/2  "Agent2"
  Bus Creator/1 -> Out1/1  "InitialConds"
  Altitude(km) Eccentricity/1 -> StartIdeal/1
  StartIdeal/1 -> Sum/2, Sum1/2, Bus Creator/3  "Agent3"

== system MultipleAgentsChoice_NoVR/StatePropagation/SatelliteControlAccel/Selective Hill State Provision and Discretisation ==
  GEOC_Current : Inport  OutDataType=sfix(16)  OutScaling=2^0
  LeadAgent : Inport  Port=2  OutDataType=sfix(16)  OutScaling=2^0
  Agent1 : Subsystem
  Agent2 : Subsystem
  Agent3 : Subsystem
  Bus Creator : BusCreator  Inputs=3
  Display{,1..3} (4 alike) : Display
  MemoryUpdate : Subsystem
  HillState : Outport  OutDataType=sfix(16)  OutScaling=2^0
  wires:
  GEOC_Current/1 -> Agent1/1(GEOC_Current), Agent2/1(GEOC_Current), Agent3/1(GEOC_Current), MemoryUpdate/1(GEOC_Current)
  LeadAgent/1 -> Agent1/2(LeadAgent), Agent2/2(LeadAgent), Agent3/2(LeadAgent), MemoryUpdate/2(LeadAgent), Display2/1
  Bus Creator/1 -> HillState/1  "HillState"
  Agent1/1(Agent1) -> Bus Creator/1, Display/1
  Agent2/1(Agent2) -> Bus Creator/2, Display1/1
  Agent3/1(Agent3) -> Bus Creator/3, Display3/1

== system MultipleAgentsChoice_NoVR/StatePropagation/SatelliteControlAccel/TriggeredSendAgent ==
  Data : Inport  OutDataType=sfix(16)  OutScaling=2^0
  Trigger : TriggerPort
  Bus Selector : BusSelector  OutputSignals=A1Data.A1ActualForces,A1Data.A1PlanMsg,A1Data.A1DesiredForces,A1Data.A1DTstate,A1Data.A1PressureData,A1Data.A1XthrusterData,A1Data.A1YthrusterData,A1Data.A1ZthrusterData,A1Data.A1XYZthrusterData,A2Data.A2ActualForces,A2Data.A2PlanMsg,A2Data.A2DesiredForces,A2Data.A2DTstate,A2Data.A2PressureData,A2Data.A2XthrusterData,A2Data.A2YthrusterData,A2Data.A2ZthrusterData,A2Data.A2XYZthrusterData,A3Data.A3ActualForces,A3Data.A3PlanMsg,A3Data.A3DesiredForces,A3Data.A3DTstate,A3Data.A3PressureData,A3Data.A3XthrusterData,A3Data.A3YthrusterData,A3Data.A3ZthrusterData,A3Data.A3XYZthrusterData
  SendToAIL : Subsystem
  wires:
  Data/1 -> Bus Selector/1
  Bus Selector/1 -> SendToAIL/1(A1ActualForces)  "<A1ActualForces>"
  Bus Selector/2 -> SendToAIL/2(A1PlanMsg)  "<A1PlanMsg>"
  Bus Selector/3 -> SendToAIL/3(A1DesiredForces)  "<A1DesiredForces>"
  Bus Selector/4 -> SendToAIL/4(A1StateInfo)  "<A1DTstate>"
  Bus Selector/6 -> SendToAIL/6(A1XThruster)  "<A1XthrusterData>"
  Bus Selector/7 -> SendToAIL/7(A1YThruster)  "<A1YthrusterData>"
  Bus Selector/8 -> SendToAIL/8(A1ZThruster)  "<A1ZthrusterData>"
  Bus Selector/9 -> SendToAIL/9(A1XYZThruster)  "<A1XYZthrusterData>"
  Bus Selector/10 -> SendToAIL/10(A2ActualForces)  "<A2ActualForces>"
  Bus Selector/11 -> SendToAIL/11(A2PlanMsg)  "<A2PlanMsg>"
  Bus Selector/12 -> SendToAIL/12(A2DesiredForces)  "<A2DesiredForces>"
  Bus Selector/13 -> SendToAIL/13(A2StateInfo)  "<A2DTstate>"
  Bus Selector/15 -> SendToAIL/15(A2XThruster)  "<A2XthrusterData>"
  Bus Selector/16 -> SendToAIL/16(A2YThruster)  "<A2YthrusterData>"
  Bus Selector/17 -> SendToAIL/17(A2ZThruster)  "<A2ZthrusterData>"
  Bus Selector/18 -> SendToAIL/18(A2XYZThruster)  "<A2XYZthrusterData>"
  Bus Selector/19 -> SendToAIL/19(A3ActualForces)  "<A3ActualForces>"
  Bus Selector/20 -> SendToAIL/20(A3PlanMsg)  "<A3PlanMsg>"
  Bus Selector/21 -> SendToAIL/21(A3DesiredForces)  "<A3DesiredForces>"
  Bus Selector/22 -> SendToAIL/22(A3StateInfo)  "<A3DTstate>"
  Bus Selector/24 -> SendToAIL/24(A3XThruster)  "<A3XthrusterData>"
  Bus Selector/25 -> SendToAIL/25(A3YThruster)  "<A3YthrusterData>"
  Bus Selector/26 -> SendToAIL/26(A3ZThruster)  "<A3ZthrusterData>"
  Bus Selector/27 -> SendToAIL/27(A3XYZThruster)  "<A3XYZthrusterData>"
  Bus Selector/5 -> SendToAIL/5(A1tank)  "<A1PressureData>"
  Bus Selector/14 -> SendToAIL/14(A2tank)  "<A2PressureData>"
  Bus Selector/23 -> SendToAIL/23(A3tank)  "<A3PressureData>"

== system MultipleAgentsChoice_NoVR/StatePropagation/SatelliteControlAccel/TriggeredSendCont ==
  Data : Inport  OutDataType=sfix(16)  OutScaling=2^0
  Trigger : TriggerPort
  Bus Selector : BusSelector  OutputSignals=A1Data.A1ActualForces,A1Data.A1PlanMsg,A1Data.A1DesiredForces,A1Data.A1DTstate,A1Data.A1PressureData,A1Data.A1XthrusterData,A1Data.A1YthrusterData,A1Data.A1ZthrusterData,A1Data.A1XYZthrusterData,A2Data.A2ActualForces,A2Data.A2PlanMsg,A2Data.A2DesiredForces,A2Data.A2DTstate,A2Data.A2PressureData,A2Data.A2XthrusterData,A2Data.A2YthrusterData,A2Data.A2ZthrusterData,A2Data.A2XYZthrusterData,A3Data.A3ActualForces,A3Data.A3PlanMsg,A3Data.A3DesiredForces,A3Data.A3DTstate,A3Data.A3PressureData,A3Data.A3XthrusterData,A3Data.A3YthrusterData,A3Data.A3ZthrusterData,A3Data.A3XYZthrusterData
  SendToCont : Subsystem
  wires:
  Bus Selector/23 -> SendToCont/23(A3tank)  "<A3PressureData>"
  Bus Selector/14 -> SendToCont/14(A2tank)  "<A2PressureData>"
  Bus Selector/5 -> SendToCont/5(A1tank)  "<A1PressureData>"
  Bus Selector/27 -> SendToCont/27(A3XYZThruster)  "<A3XYZthrusterData>"
  Bus Selector/26 -> SendToCont/26(A3ZThruster)  "<A3ZthrusterData>"
  Bus Selector/25 -> SendToCont/25(A3YThruster)  "<A3YthrusterData>"
  Bus Selector/24 -> SendToCont/24(A3XThruster)  "<A3XthrusterData>"
  Bus Selector/22 -> SendToCont/22(A3StateInfo)  "<A3DTstate>"
  Bus Selector/21 -> SendToCont/21(A3DesiredForces)  "<A3DesiredForces>"
  Bus Selector/20 -> SendToCont/20(A3PlanMsg)  "<A3PlanMsg>"
  Bus Selector/19 -> SendToCont/19(A3ActualForces)  "<A3ActualForces>"
  Bus Selector/18 -> SendToCont/18(A2XYZThruster)  "<A2XYZthrusterData>"
  Bus Selector/17 -> SendToCont/17(A2ZThruster)  "<A2ZthrusterData>"
  Bus Selector/16 -> SendToCont/16(A2YThruster)  "<A2YthrusterData>"
  Bus Selector/15 -> SendToCont/15(A2XThruster)  "<A2XthrusterData>"
  Bus Selector/13 -> SendToCont/13(A2StateInfo)  "<A2DTstate>"
  Bus Selector/12 -> SendToCont/12(A2DesiredForces)  "<A2DesiredForces>"
  Bus Selector/11 -> SendToCont/11(A2PlanMsg)  "<A2PlanMsg>"
  Bus Selector/10 -> SendToCont/10(A2ActualForces)  "<A2ActualForces>"
  Bus Selector/9 -> SendToCont/9(A1XYZThruster)  "<A1XYZthrusterData>"
  Bus Selector/8 -> SendToCont/8(A1ZThruster)  "<A1ZthrusterData>"
  Bus Selector/7 -> SendToCont/7(A1YThruster)  "<A1YthrusterData>"
  Bus Selector/6 -> SendToCont/6(A1XThruster)  "<A1XthrusterData>"
  Bus Selector/4 -> SendToCont/4(A1StateInfo)  "<A1DTstate>"
  Bus Selector/3 -> SendToCont/3(A1DesiredForces)  "<A1DesiredForces>"
  Bus Selector/2 -> SendToCont/2(A1PlanMsg)  "<A1PlanMsg>"
  Bus Selector/1 -> SendToCont/1(A1ActualForces)  "<A1ActualForces>"
  Data/1 -> Bus Selector/1

== system MultipleAgentsChoice_NoVR/RealTime/Real-time synchronization/Real-time Synchronization/Subsystem ==
  In : Inport
  Trigger : TriggerPort
  Out : Outport  InitialOutput=0
  wires:
  In/1 -> Out/1

== system MultipleAgentsChoice_NoVR/StatePropagation/BodyAccelerations/Agent1/EarthAccel(J2) ==
  JT : Inport  OutDataType=sfix(16)  OutScaling=2^0
  GEOC_Pos : Inport  Port=2  OutDataType=sfix(16)  OutScaling=2^0
  MultiOrderEarthJ2 function : MATLABFcn  MATLABFcn=MultiOrderEarthJ2  OutputDimensions=3
  Mux : Mux  Inputs=2
  AccelEarth : Outport  OutDataType=sfix(16)  OutScaling=2^0
  wires:
  MultiOrderEarthJ2 function/1 -> AccelEarth/1
  JT/1 -> Mux/1
  GEOC_Pos/1 -> Mux/2
  Mux/1 -> MultiOrderEarthJ2 function/1

== system MultipleAgentsChoice_NoVR/StatePropagation/BodyAccelerations/Agent1/EarthAccel1 ==
  GEOC_Pos : Inport  OutDataType=sfix(16)  OutScaling=2^0
  EarthJ2 function : MATLABFcn  MATLABFcn=TwoBodyEarth
  AccelEarth : Outport  OutDataType=sfix(16)  OutScaling=2^0
  wires:
  GEOC_Pos/1 -> EarthJ2 function/1
  EarthJ2 function/1 -> AccelEarth/1

== system MultipleAgentsChoice_NoVR/StatePropagation/BodyAccelerations/Agent1/MoonAccel ==
  JT : Inport  OutDataType=sfix(16)  OutScaling=2^0
  SatGEOC_Pos : Inport  Port=2  OutDataType=sfix(16)  OutScaling=2^0
  MoonCalc1 : MATLABFcn  MATLABFcn=MoonCalc
  MoonDirVector : MATLABFcn  MATLABFcn=moon
  Mux : Mux  Inputs=2
  Re : Gain  Gain=6371  ParameterDataType=sfix(16)  ParameterScaling=2^0  OutDataType=sfix(16)  OutScaling=2^0
  AccelMoon : Outport  OutDataType=sfix(16)  OutScaling=2^0
  wires:
  JT/1 -> MoonDirVector/1
  MoonDirVector/1 -> Re/1
  Re/1 -> Mux/2
  SatGEOC_Pos/1 -> Mux/1
  MoonCalc1/1 -> AccelMoon/1
  Mux/1 -> MoonCalc1/1

== system MultipleAgentsChoice_NoVR/StatePropagation/BodyAccelerations/Agent1/SRPAccel ==
  JT1 : Inport  OutDataType=sfix(16)  OutScaling=2^0
  GEOC_Pos1 : Inport  Port=2  OutDataType=sfix(16)  OutScaling=2^0
  AU : Gain  Gain=1.4960e8  ParameterDataType=sfix(16)  ParameterScaling=2^0  OutDataType=sfix(16)  OutScaling=2^0
  Mux : Mux  Inputs=2
  SRPCalc : MATLABFcn  MATLABFcn=SRPCalc
  SRPF : Constant  Value=1e-6  OutDataType=sfix(16)  OutScaling=2^0
  Sum : Sum  Inputs=|+-  OutDataType=sfix(16)  OutScaling=2^0
  SunDirVector : MATLABFcn  MATLABFcn=sun
  AccelSRP : Outport  OutDataType=sfix(16)  OutScaling=2^0
  wires:
  JT1/1 -> SunDirVector/1
  SunDirVector/1 -> AU/1
  SRPCalc/1 -> AccelSRP/1
  SRPF/1 -> Mux/2
  Mux/1 -> SRPCalc/1
  AU/1 -> Sum/1
  Sum/1 -> Mux/1
  GEOC_Pos1/1 -> Sum/2

== system MultipleAgentsChoice_NoVR/StatePropagation/BodyAccelerations/Agent1/SunAccel ==
  JT1 : Inport  OutDataType=sfix(16)  OutScaling=2^0
  SatGEOC_Pos1 : Inport  Port=2  OutDataType=sfix(16)  OutScaling=2^0
  AU : Gain  Gain=1.4960e8  ParameterDataType=sfix(16)  ParameterScaling=2^0  OutDataType=sfix(16)  OutScaling=2^0
  Mux : Mux  Inputs=2
  SunAccel : MATLABFcn  MATLABFcn=SunCalc
  SunDirVector : MATLABFcn  MATLABFcn=sun
  AccelSun : Outport  OutDataType=sfix(16)  OutScaling=2^0
  wires:
  JT1/1 -> SunDirVector/1
  SunDirVector/1 -> AU/1
  SunAccel/1 -> AccelSun/1
  Mux/1 -> SunAccel/1
  SatGEOC_Pos1/1 -> Mux/1
  AU/1 -> Mux/2

== system MultipleAgentsChoice_NoVR/StatePropagation/BodyAccelerations/Agent2/EarthAccel(J2) ==
  JT : Inport  OutDataType=sfix(16)  OutScaling=2^0
  GEOC_Pos : Inport  Port=2  OutDataType=sfix(16)  OutScaling=2^0
  MultiOrderEarthJ2 function : MATLABFcn  MATLABFcn=MultiOrderEarthJ2  OutputDimensions=3
  Mux : Mux  Inputs=2
  AccelEarth : Outport  OutDataType=sfix(16)  OutScaling=2^0
  wires:
  Mux/1 -> MultiOrderEarthJ2 function/1
  GEOC_Pos/1 -> Mux/2
  JT/1 -> Mux/1
  MultiOrderEarthJ2 function/1 -> AccelEarth/1

== system MultipleAgentsChoice_NoVR/StatePropagation/BodyAccelerations/Agent2/EarthAccel1 ==
  GEOC_Pos : Inport  OutDataType=sfix(16)  OutScaling=2^0
  EarthJ2 function : MATLABFcn  MATLABFcn=TwoBodyEarth
  AccelEarth : Outport  OutDataType=sfix(16)  OutScaling=2^0
  wires:
  EarthJ2 function/1 -> AccelEarth/1
  GEOC_Pos/1 -> EarthJ2 function/1

== system MultipleAgentsChoice_NoVR/StatePropagation/BodyAccelerations/Agent2/MoonAccel ==
  JT : Inport  OutDataType=sfix(16)  OutScaling=2^0
  SatGEOC_Pos : Inport  Port=2  OutDataType=sfix(16)  OutScaling=2^0
  MoonCalc1 : MATLABFcn  MATLABFcn=MoonCalc
  MoonDirVector : MATLABFcn  MATLABFcn=moon
  Mux : Mux  Inputs=2
  Re : Gain  Gain=6371  ParameterDataType=sfix(16)  ParameterScaling=2^0  OutDataType=sfix(16)  OutScaling=2^0
  AccelMoon : Outport  OutDataType=sfix(16)  OutScaling=2^0
  wires:
  Mux/1 -> MoonCalc1/1
  MoonCalc1/1 -> AccelMoon/1
  SatGEOC_Pos/1 -> Mux/1
  Re/1 -> Mux/2
  MoonDirVector/1 -> Re/1
  JT/1 -> MoonDirVector/1

== system MultipleAgentsChoice_NoVR/StatePropagation/BodyAccelerations/Agent2/SRPAccel ==
  JT1 : Inport  OutDataType=sfix(16)  OutScaling=2^0
  GEOC_Pos1 : Inport  Port=2  OutDataType=sfix(16)  OutScaling=2^0
  AU : Gain  Gain=1.4960e8  ParameterDataType=sfix(16)  ParameterScaling=2^0  OutDataType=sfix(16)  OutScaling=2^0
  Mux : Mux  Inputs=2
  SRPCalc : MATLABFcn  MATLABFcn=SRPCalc
  SRPF : Constant  Value=1e-6  OutDataType=sfix(16)  OutScaling=2^0
  Sum : Sum  Inputs=|+-  OutDataType=sfix(16)  OutScaling=2^0
  SunDirVector : MATLABFcn  MATLABFcn=sun
  AccelSRP : Outport  OutDataType=sfix(16)  OutScaling=2^0
  wires:
  GEOC_Pos1/1 -> Sum/2
  Sum/1 -> Mux/1
  AU/1 -> Sum/1
  Mux/1 -> SRPCalc/1
  SRPF/1 -> Mux/2
  SRPCalc/1 -> AccelSRP/1
  SunDirVector/1 -> AU/1
  JT1/1 -> SunDirVector/1

== system MultipleAgentsChoice_NoVR/StatePropagation/BodyAccelerations/Agent2/SunAccel ==
  JT1 : Inport  OutDataType=sfix(16)  OutScaling=2^0
  SatGEOC_Pos1 : Inport  Port=2  OutDataType=sfix(16)  OutScaling=2^0
  AU : Gain  Gain=1.4960e8  ParameterDataType=sfix(16)  ParameterScaling=2^0  OutDataType=sfix(16)  OutScaling=2^0
  Mux : Mux  Inputs=2
  SunAccel : MATLABFcn  MATLABFcn=SunCalc
  SunDirVector : MATLABFcn  MATLABFcn=sun
  AccelSun : Outport  OutDataType=sfix(16)  OutScaling=2^0
  wires:
  AU/1 -> Mux/2
  SatGEOC_Pos1/1 -> Mux/1
  Mux/1 -> SunAccel/1
  SunAccel/1 -> AccelSun/1
  SunDirVector/1 -> AU/1
  JT1/1 -> SunDirVector/1

== system MultipleAgentsChoice_NoVR/StatePropagation/BodyAccelerations/Agent3/EarthAccel(J2) ==
  JT : Inport  OutDataType=sfix(16)  OutScaling=2^0
  GEOC_Pos : Inport  Port=2  OutDataType=sfix(16)  OutScaling=2^0
  MultiOrderEarthJ2 function : MATLABFcn  MATLABFcn=MultiOrderEarthJ2  OutputDimensions=3
  Mux : Mux  Inputs=2
  AccelEarth : Outport  OutDataType=sfix(16)  OutScaling=2^0
  wires:
  MultiOrderEarthJ2 function/1 -> AccelEarth/1
  JT/1 -> Mux/1
  GEOC_Pos/1 -> Mux/2
  Mux/1 -> MultiOrderEarthJ2 function/1

== system MultipleAgentsChoice_NoVR/StatePropagation/BodyAccelerations/Agent3/EarthAccel1 ==
  GEOC_Pos : Inport  OutDataType=sfix(16)  OutScaling=2^0
  EarthJ2 function : MATLABFcn  MATLABFcn=TwoBodyEarth
  AccelEarth : Outport  OutDataType=sfix(16)  OutScaling=2^0
  wires:
  GEOC_Pos/1 -> EarthJ2 function/1
  EarthJ2 function/1 -> AccelEarth/1

== system MultipleAgentsChoice_NoVR/StatePropagation/BodyAccelerations/Agent3/MoonAccel ==
  JT : Inport  OutDataType=sfix(16)  OutScaling=2^0
  SatGEOC_Pos : Inport  Port=2  OutDataType=sfix(16)  OutScaling=2^0
  MoonCalc1 : MATLABFcn  MATLABFcn=MoonCalc
  MoonDirVector : MATLABFcn  MATLABFcn=moon
  Mux : Mux  Inputs=2
  Re : Gain  Gain=6371  ParameterDataType=sfix(16)  ParameterScaling=2^0  OutDataType=sfix(16)  OutScaling=2^0
  AccelMoon : Outport  OutDataType=sfix(16)  OutScaling=2^0
  wires:
  JT/1 -> MoonDirVector/1
  MoonDirVector/1 -> Re/1
  Re/1 -> Mux/2
  SatGEOC_Pos/1 -> Mux/1
  MoonCalc1/1 -> AccelMoon/1
  Mux/1 -> MoonCalc1/1

== system MultipleAgentsChoice_NoVR/StatePropagation/BodyAccelerations/Agent3/SRPAccel ==
  JT1 : Inport  OutDataType=sfix(16)  OutScaling=2^0
  GEOC_Pos1 : Inport  Port=2  OutDataType=sfix(16)  OutScaling=2^0
  AU : Gain  Gain=1.4960e8  ParameterDataType=sfix(16)  ParameterScaling=2^0  OutDataType=sfix(16)  OutScaling=2^0
  Mux : Mux  Inputs=2
  SRPCalc : MATLABFcn  MATLABFcn=SRPCalc
  SRPF : Constant  Value=1e-6  OutDataType=sfix(16)  OutScaling=2^0
  Sum : Sum  Inputs=|+-  OutDataType=sfix(16)  OutScaling=2^0
  SunDirVector : MATLABFcn  MATLABFcn=sun
  AccelSRP : Outport  OutDataType=sfix(16)  OutScaling=2^0
  wires:
  JT1/1 -> SunDirVector/1
  SunDirVector/1 -> AU/1
  SRPCalc/1 -> AccelSRP/1
  SRPF/1 -> Mux/2
  Mux/1 -> SRPCalc/1
  AU/1 -> Sum/1
  Sum/1 -> Mux/1
  GEOC_Pos1/1 -> Sum/2

== system MultipleAgentsChoice_NoVR/StatePropagation/BodyAccelerations/Agent3/SunAccel ==
  JT1 : Inport  OutDataType=sfix(16)  OutScaling=2^0
  SatGEOC_Pos1 : Inport  Port=2  OutDataType=sfix(16)  OutScaling=2^0
  AU : Gain  Gain=1.4960e8  ParameterDataType=sfix(16)  ParameterScaling=2^0  OutDataType=sfix(16)  OutScaling=2^0
  Mux : Mux  Inputs=2
  SunAccel : MATLABFcn  MATLABFcn=SunCalc
  SunDirVector : MATLABFcn  MATLABFcn=sun
  AccelSun : Outport  OutDataType=sfix(16)  OutScaling=2^0
  wires:
  JT1/1 -> SunDirVector/1
  SunDirVector/1 -> AU/1
  SunAccel/1 -> AccelSun/1
  Mux/1 -> SunAccel/1
  SatGEOC_Pos1/1 -> Mux/1
  AU/1 -> Mux/2
